simulink model "ISRTest2"  (Simulink 6.6)
settings: Solver=ode3  StartTime=0.0  StopTime=time(end)  FixedStep=0.01  RelTol=1e-3
values from neighbouring files (symbols this model uses):
  apSampleTime = 0.01    [Load_Replay.m]    (also in loadReplayMay2013.m; loadTuneRollReplay_May2013.m; replayFlight.m)
  bankCommandLimit = single(45*pi/180)    [replayFlight.m]
  ISA_g = 9.815    [replayFlight.m]
undefined symbols (not defined in the file or in its folder): fOrderingInOut, maxAcc, maxEta
libraries: simulink x14, aerolibconvert2 x11, dsPICdrivers x7, SLUGS_Library x3, dspmtrx3 x2, aerolibutil x1
(part 1 of 2)
settings Model: Creator=Administrator  LastModifiedBy=Administrator

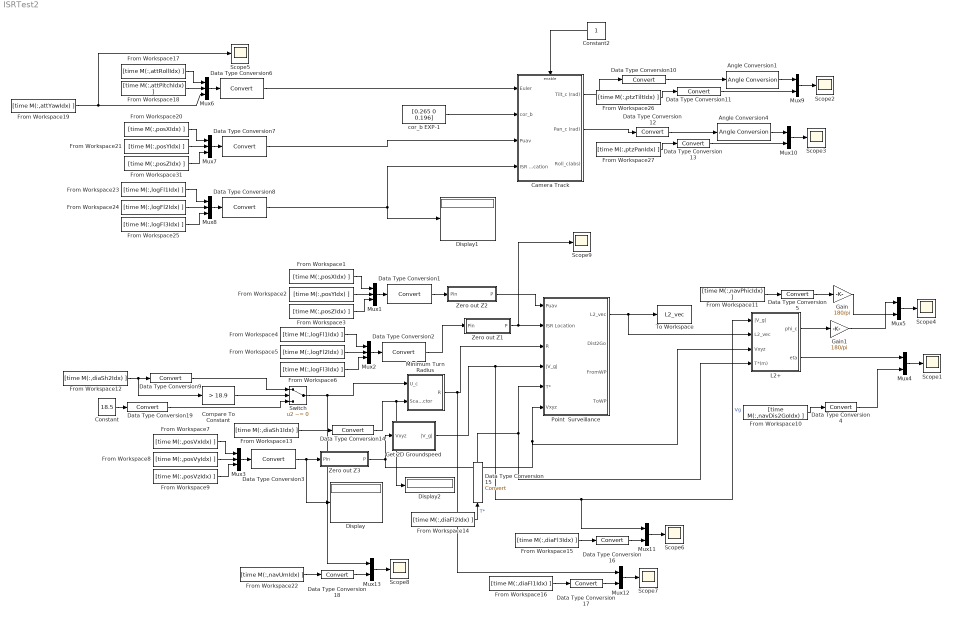
== system ISRTest2 ==
  Angle Conversion1 : aerolibconvert2/Angle Conversion  SystemSampleTime=-1  IU=rad  OU=deg
  Angle Conversion4 : aerolibconvert2/Angle Conversion  SystemSampleTime=-1  IU=rad  OU=deg
  Camera Track : Subsystem  TreatAsAtomicUnit=on  SystemSampleTime=0.01
  Compare To Constant : simulink/Logic and Bit Operations/Compare To Constant  SystemSampleTime=-1  relop=>  const=18.9  LogicOutDataTypeMode=uint8  ZeroCross=off
  Constant : Constant  Value=18.5
  Constant2 : Constant  Orientation=left  OutDataTypeMode=uint8
  Data Type Conversion{1..14,16..19} (18 alike) : DataTypeConversion  OutDataTypeMode=single
  Data Type Conversion15 : DataTypeConversion  Orientation=up  OutDataTypeMode=single
  Display : Display
  Display1 : Display
  Display2 : Display
  From Workspace1 : FromWorkspace  VariableName=[time M(:,posXIdx) ]  SampleTime=0.01
  From Workspace10 : FromWorkspace  VariableName=[time M(:,navDis2GoIdx) ]  SampleTime=0.01
  From Workspace11 : FromWorkspace  VariableName=[time M(:,navPhicIdx) ]  SampleTime=0.01
  From Workspace12 : FromWorkspace  VariableName=[time M(:,diaSh2Idx) ]  SampleTime=0.01
  From Workspace13 : FromWorkspace  VariableName=[time M(:,diaSh1Idx) ]  SampleTime=0.01
  From Workspace14 : FromWorkspace  VariableName=[time M(:,diaFl2Idx) ]  SampleTime=0.01
  From Workspace15 : FromWorkspace  VariableName=[time M(:,diaFl3Idx) ]  SampleTime=0.01
  From Workspace16 : FromWorkspace  VariableName=[time M(:,diaFl1Idx) ]  SampleTime=0.01
  From Workspace17 : FromWorkspace  VariableName=[time M(:,attRollIdx) ]  SampleTime=0.01
  From Workspace18 : FromWorkspace  VariableName=[time M(:,attPitchIdx) ]  SampleTime=0.01
  From Workspace19 : FromWorkspace  VariableName=[time M(:,attYawIdx) ]  SampleTime=0.01
  From Workspace2 : FromWorkspace  VariableName=[time M(:,posYIdx) ]  SampleTime=0.01
  From Workspace20 : FromWorkspace  VariableName=[time M(:,posXIdx) ]  SampleTime=0.01
  From Workspace21 : FromWorkspace  VariableName=[time M(:,posYIdx) ]  SampleTime=0.01
  From Workspace22 : FromWorkspace  VariableName=[time M(:,navUmIdx) ]  SampleTime=0.01
  From Workspace23 : FromWorkspace  VariableName=[time M(:,logFl1Idx) ]  SampleTime=0.01
  From Workspace24 : FromWorkspace  VariableName=[time M(:,logFl2Idx) ]  SampleTime=0.01
  From Workspace25 : FromWorkspace  VariableName=[time M(:,logFl3Idx) ]  SampleTime=0.01
  From Workspace26 : FromWorkspace  VariableName=[time M(:,ptzTiltIdx) ]  SampleTime=0.01
  From Workspace27 : FromWorkspace  VariableName=[time M(:,ptzPanIdx) ]  SampleTime=0.01
  From Workspace3 : FromWorkspace  VariableName=[time M(:,posZIdx) ]  SampleTime=0.01
  From Workspace31 : FromWorkspace  VariableName=[time M(:,posZIdx) ]  SampleTime=0.01
  From Workspace4 : FromWorkspace  VariableName=[time M(:,logFl1Idx) ]  SampleTime=0.01
  From Workspace5 : FromWorkspace  VariableName=[time M(:,logFl2Idx) ]  SampleTime=0.01
  From Workspace6 : FromWorkspace  VariableName=[time M(:,logFl3Idx) ]  SampleTime=0.01
  From Workspace7 : FromWorkspace  VariableName=[time M(:,posVxIdx) ]  SampleTime=0.01
  From Workspace8 : FromWorkspace  VariableName=[time M(:,posVyIdx) ]  SampleTime=0.01
  From Workspace9 : FromWorkspace  VariableName=[time M(:,posVzIdx) ]  SampleTime=0.01
  Gain : Gain  Gain=180/pi
  Gain1 : Gain  Gain=180/pi
  Get 2D Groundspeed : Subsystem
  L2+ : Subsystem
  Minimum Turn Radius : Subsystem
  Mux{1..3,6..8} (6 alike) : Mux  Inputs=3
  Mux{4..5,9..13} (7 alike) : Mux  Inputs=2
  Point  Surveillance : Subsystem  TreatAsAtomicUnit=on
  Scope{1..9} (9 alike) : Scope
      Scope1 settings: YMin=-120  YMax=30
      Scope2 settings: TimeRange=1267.6  YMin=-65  YMax=0  SaveName=ScopeData5
      Scope3 settings: TimeRange=600  YMin=49.80645682246021  YMax=134.5919948321196  SaveName=ScopeData6
      Scope4 settings: YMin=-15  YMax=25  SaveName=ScopeData7
      Scope5 settings: SaveName=ScopeData10
      Scope6 settings: TimeRange=600  YMin=12  YMax=24  SaveName=ScopeData11
      Scope7 settings: YMin=373  YMax=395  SaveName=ScopeData12
      Scope8 settings: YMin=17.75  YMax=20.25  SaveName=ScopeData13
      Scope9 settings: TimeRange=1429.39  YMin=-67.5  YMax=-27.5  SaveName=ScopeData19
  Switch : Switch  Criteria=u2 ~= 0  Threshold=0.3
  To Workspace : ToWorkspace  VariableName=L2_vec  SampleTime=-1  SaveFormat=Array
  Zero out Z1 : Stateflow chart
  Zero out Z2 : Stateflow chart
  Zero out Z3 : Stateflow chart
  cor_b EXP-1 : Constant  Value=[0.265 0 0.196]  OutDataTypeMode=single
  wires:
  Mux6/1 -> Data Type Conversion6/1
  From Workspace17/1 -> Mux6/1
  From Workspace18/1 -> Mux6/2
  From Workspace19/1 -> Mux6/3, Scope5/1
  Data Type Conversion6/1 -> Camera Track/1(Euler)
  cor_b EXP-1/1 -> Camera Track/2(cor_b)
  Mux7/1 -> Data Type Conversion7/1
  From Workspace20/1 -> Mux7/1
  From Workspace21/1 -> Mux7/2
  Data Type Conversion7/1 -> Camera Track/3(Puav)
  Mux8/1 -> Data Type Conversion8/1
  From Workspace23/1 -> Mux8/1
  From Workspace24/1 -> Mux8/2
  From Workspace25/1 -> Mux8/3
  Data Type Conversion8/1 -> Camera Track/4(ISR Location), Display1/1
  Constant2/1 -> Camera Track/Enable
  Mux9/1 -> Scope2/1
  Camera Track/1(Tilt_c (rad)) -> Data Type Conversion10/1
  From Workspace26/1 -> Data Type Conversion11/1
  Mux10/1 -> Scope3/1
  From Workspace27/1 -> Data Type Conversion13/1
  Camera Track/2(Pan_c (rad)) -> Data Type Conversion12/1
  Data Type Conversion10/1 -> Angle Conversion1/1
  Data Type Conversion11/1 -> Mux9/2
  Data Type Conversion12/1 -> Angle Conversion4/1
  Data Type Conversion13/1 -> Mux10/2
  From Workspace31/1 -> Mux7/3
  Angle Conversion4/1 -> Mux10/1
  Angle Conversion1/1 -> Mux9/1
  Mux1/1 -> Data Type Conversion1/1
  From Workspace1/1 -> Mux1/1
  From Workspace2/1 -> Mux1/2
  From Workspace3/1 -> Mux1/3
  Data Type Conversion1/1 -> Zero out Z2/1(Pin)
  Zero out Z2/1(P) -> Point  Surveillance/1(Puav)
  Mux2/1 -> Data Type Conversion2/1
  From Workspace4/1 -> Mux2/1
  From Workspace5/1 -> Mux2/2
  From Workspace6/1 -> Mux2/3
  Data Type Conversion2/1 -> Zero out Z1/1(Pin)
  Zero out Z1/1(P) -> Point  Surveillance/2(ISR Location), Scope9/1
  Minimum Turn Radius/1(R) -> Point  Surveillance/3(R), Mux12/1
  From Workspace12/1 -> Data Type Conversion9/1, Compare To Constant/1
  From Workspace13/1 -> Data Type Conversion14/1
  Zero out Z3/1(P) -> Get 2D Groundspeed/1(Vxyz), L2+/3(Vxyz), Point  Surveillance/6(Vxyz)
  Get 2D Groundspeed/1(|V_g|) -> Point  Surveillance/4(|V_g|), L2+/1(|V_g|), Mux11/1  "Vg"
  Mux3/1 -> Data Type Conversion3/1
  From Workspace7/1 -> Mux3/1
  From Workspace8/1 -> Mux3/2
  From Workspace9/1 -> Mux3/3
  Data Type Conversion3/1 -> Zero out Z3/1(Pin), Display/1
  From Workspace14/1 -> Data Type Conversion15/1  "T*"
  Point  Surveillance/1(L2_vec) -> To Workspace/1, L2+/2(L2_vec)
  L2+/2(eta) -> Mux4/1
  Mux4/1 -> Scope1/1
  From Workspace10/1 -> Data Type Conversion4/1
  Data Type Conversion4/1 -> Mux4/2
  Mux5/1 -> Scope4/1
  From Workspace11/1 -> Data Type Conversion5/1
  Data Type Conversion5/1 -> Gain/1
  L2+/1(phi_c) -> Gain1/1
  Data Type Conversion14/1 -> Minimum Turn Radius/2(Scale Factor), Display2/1
  Data Type Conversion15/1 -> L2+/4(T*(m)), Point  Surveillance/5(T*)
  Gain/1 -> Mux5/2
  Gain1/1 -> Mux5/1
  Mux11/1 -> Scope6/1
  From Workspace15/1 -> Data Type Conversion16/1
  Data Type Conversion16/1 -> Mux11/2
  Mux12/1 -> Scope7/1
  From Workspace16/1 -> Data Type Conversion17/1
  Data Type Conversion17/1 -> Mux12/2
  From Workspace22/1 -> Data Type Conversion18/1
  Data Type Conversion18/1 -> Mux13/2
  Mux13/1 -> Scope8/1
  Switch/1 -> Minimum Turn Radius/1(U_c), Mux13/1
  Data Type Conversion9/1 -> Switch/1
  Compare To Constant/1 -> Switch/2
  Constant/1 -> Data Type Conversion19/1
  Data Type Conversion19/1 -> Switch/3

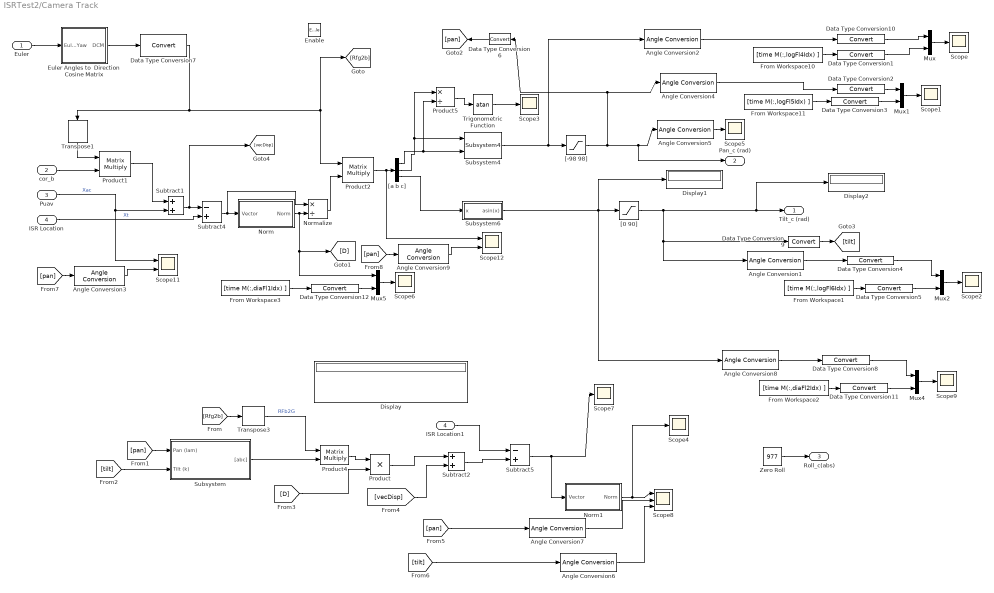
== system ISRTest2/Camera Track ==
  Euler : Inport
  cor_b : Inport  Port=2
  Puav : Inport  Port=3
  ISR Location : Inport  Port=4
  Enable : EnablePort
  Angle Conversion{1..9} (9 alike) : aerolibconvert2/Angle Conversion  SystemSampleTime=-1  IU=rad  OU=deg
  Data Type Conversion{1..5,7..12} (11 alike) : DataTypeConversion  OutDataTypeMode=single
  Data Type Conversion6 : DataTypeConversion  Orientation=left  OutDataTypeMode=single
  Display : Display
  Display1 : Display
  Display2 : Display
  Euler Angles to  Direction Cosine Matrix : Subsystem  AncestorBlock="aerolibtransform2/Euler Angles to  Direction Cosine Matrix"  mask(Euler2DCM){}
      mask help: Determine the 3-by-3 direction cosine matrix (DCM) from an Euler orientation (roll, pitch, yaw). The output DCM transforms vectors from geodetic earth or north-east-down (NED) axes to body axes.
      mask init:
      | aeroicon('aeroblk');
      mask Help: web(asbhelp('euleranglestodirectioncosinematrix'));
      mask Display:
      | port_label('input',1,'\phi \theta \psi','texmode','on')
      | port_label('output',1,'DCM_{be}','texmode','on')
  From Workspace1 : FromWorkspace  VariableName=[time M(:,logFl6Idx) ]  SampleTime=0.01
  From Workspace10 : FromWorkspace  VariableName=[time M(:,logFl4Idx) ]  SampleTime=0.01
  From Workspace11 : FromWorkspace  VariableName=[time M(:,logFl5Idx) ]  SampleTime=0.01
  From Workspace2 : FromWorkspace  VariableName=[time M(:,diaFl2Idx) ]  SampleTime=0.01
  From Workspace3 : FromWorkspace  VariableName=[time M(:,diaFl1Idx) ]  SampleTime=0.01
  ISR Location1 : InportShadow  Port=4  LatchByCopyingInsideSignal=off
  Mux{,1..2,4..5} (5 alike) : Mux  Inputs=2
  Norm : Subsystem
  Norm1 : Subsystem
  Normalize : Product  Inputs=*/  OutScaling=2^-10
  Product : Product  RndMeth=Zero
  Product1 : Product  Multiplication=Matrix(*)  RndMeth=Zero
  Product2 : Product  Multiplication=Matrix(*)  RndMeth=Zero
  Product4 : Product  Multiplication=Matrix(*)  RndMeth=Zero
  Product5 : Product  Inputs=*/  RndMeth=Zero
  Scope{,1..7,9} (9 alike) : Scope
      Scope settings: YMin=20  YMax=170  SaveName=ScopeData2
      Scope1 settings: SaveName=ScopeData3
      Scope2 settings: SaveName=ScopeData4
      Scope3 settings: YMin=-1.75  YMax=1.75  SaveName=ScopeData8
      Scope4 settings: YMin=0  YMax=75
      Scope5 settings: YMin=-90  YMax=90  SaveName=ScopeData14
      Scope6 settings: YMin=-90  YMax=90  SaveName=ScopeData15
      Scope7 settings: YMin=-90  YMax=90  SaveName=ScopeData16
      Scope9 settings: SaveName=ScopeData18
  Scope11 : Scope  NumInputPorts=2
      settings: YMin=-125~-100  YMax=175~100  SaveName=ScopeData20
  Scope12 : Scope  NumInputPorts=2
      settings: YMin=-1~-57.5  YMax=0.4~-20  SaveName=ScopeData21
  Scope8 : Scope  NumInputPorts=3
      settings: YMin=0~-100~57.5  YMax=110~100~90  SaveName=ScopeData17
  Subsystem : Subsystem
  Subsystem4 : SLUGS_Library/Subsystem4  SystemSampleTime=-1
  Subsystem6 : Subsystem  AncestorBlock=SLUGS_Library/Subsystem6
  Subtract1 : Sum  OutScaling=2^-10
  Subtract2 : Sum  OutScaling=2^-10
  Subtract4 : Sum  Inputs=-+  OutScaling=2^-10
  Subtract5 : Sum  Inputs=-+  OutScaling=2^-10
  Transpose1 : dspmtrx3/Transpose  Orientation=down  SystemSampleTime=-1  Hermitian=off  overflowFlag=off
  Transpose3 : dspmtrx3/Transpose  SystemSampleTime=-1  Hermitian=off  overflowFlag=off
  Trigonometric Function : Trigonometry  Operator=atan
  Zero Roll : Constant  Value=977  OutDataTypeMode=uint16
  "[-98 98]" : Saturate  UpperLimit=1.7104  LowerLimit=-1.7104
  "[0 90]" : Saturate  UpperLimit=0  LowerLimit=-pi/2
  "[a b c]" : Demux  Outputs=3
  Tilt_c (rad) : Outport
  Pan_c (rad) : Outport  Port=2
  Roll_c(abs) : Outport  Port=3  InitialOutput=977
  wires:
  Angle Conversion1/1 -> Data Type Conversion4/1
  Angle Conversion2/1 -> Data Type Conversion10/1
  Zero Roll/1 -> Roll_c(abs)/1
  cor_b/1 -> Product1/2
  Norm/1(Norm) -> Normalize/2, [D], Mux5/1
  Normalize/1 -> Product2/2
  Product2/1 -> "[a b c]"/1, Scope12/1
  "[a b c]"/3 -> Subsystem6/1(x)
  "[a b c]"/2 -> Subsystem4/1, Product5/1
  "[a b c]"/1 -> Subsystem4/2, Product5/2
  Subtract4/1 -> Norm/1(Vector), Normalize/1
  "[0 90]"/1 -> Angle Conversion1/1, Data Type Conversion9/1, Tilt_c (rad)/1, Display2/1
  Mux/1 -> Scope/1
  From Workspace10/1 -> Data Type Conversion1/1
  Mux1/1 -> Scope1/1
  Angle Conversion4/1 -> Data Type Conversion2/1
  From Workspace11/1 -> Data Type Conversion3/1
  Mux2/1 -> Scope2/1
  From Workspace1/1 -> Data Type Conversion5/1
  Data Type Conversion10/1 -> Mux/1
  Data Type Conversion1/1 -> Mux/2
  Data Type Conversion2/1 -> Mux1/1
  Data Type Conversion3/1 -> Mux1/2
  Data Type Conversion4/1 -> Mux2/1
  Data Type Conversion5/1 -> Mux2/2
  Transpose1/1 -> Product1/1
  Subtract1/1 -> Subtract4/1, [vecDisp]
  ISR Location/1 -> Subtract4/2  "Xt"
  Product1/1 -> Subtract1/1
  Puav/1 -> Subtract1/2, Scope11/1  "Xac"
  Subsystem4/1 -> "[-98 98]"/1, Angle Conversion2/1
  Angle Conversion5/1 -> Scope5/1
  "[-98 98]"/1 -> Data Type Conversion6/1, Angle Conversion4/1, Angle Conversion5/1, Pan_c (rad)/1
  Data Type Conversion9/1 -> [tilt]
  Data Type Conversion6/1 -> [pan]
  [Rfg2b] -> Transpose3/1
  Subsystem/1("[abc]") -> Product4/2
  Transpose3/1 -> Product4/1  "RFb2G"
  [vecDisp] -> Subtract2/2
  Subtract2/1 -> Subtract5/2
  ISR Location1/1 -> Subtract5/1
  Subtract5/1 -> Scope7/1, Norm1/1(Vector)
  Norm1/1(Norm) -> Scope8/1, Scope4/1
  [pan] -> Angle Conversion7/1
  Angle Conversion7/1 -> Scope8/2
  Angle Conversion6/1 -> Scope8/3
  Euler Angles to  Direction Cosine Matrix/1(DCM) -> Data Type Conversion7/1
  Euler/1 -> Euler Angles to  Direction Cosine Matrix/1(Euler Roll Pitch Yaw)
  Data Type Conversion7/1 -> Transpose1/1, Product2/1, [Rfg2b]
  Subsystem6/1(asin(x)) -> Angle Conversion8/1, Display1/1, "[0 90]"/1
  Angle Conversion8/1 -> Data Type Conversion8/1
  Mux4/1 -> Scope9/1
  From Workspace2/1 -> Data Type Conversion11/1
  Data Type Conversion8/1 -> Mux4/1
  Data Type Conversion11/1 -> Mux4/2
  From Workspace3/1 -> Data Type Conversion12/1
  Data Type Conversion12/1 -> Mux5/2
  Mux5/1 -> Scope6/1
  Trigonometric Function/1 -> Scope3/1
  [pan] -> Angle Conversion3/1
  Angle Conversion3/1 -> Scope11/2
  [pan] -> Angle Conversion9/1
  Angle Conversion9/1 -> Scope12/2
  [tilt] -> Angle Conversion6/1
  Product5/1 -> Trigonometric Function/1
  Product4/1 -> Product/1
  [D] -> Product/2
  Product/1 -> Subtract2/1
  [pan] -> Subsystem/1(Pan (lam))
  [tilt] -> Subsystem/2(Tilt (k))

== system ISRTest2/Get 2D Groundspeed ==
  Vxyz : Inport  SampleTime=apSampleTime
  Norm : Subsystem
  |V_g| : Outport
  wires:
  Norm/1(Norm) -> |V_g|/1
  Vxyz/1 -> Norm/1(Vector)

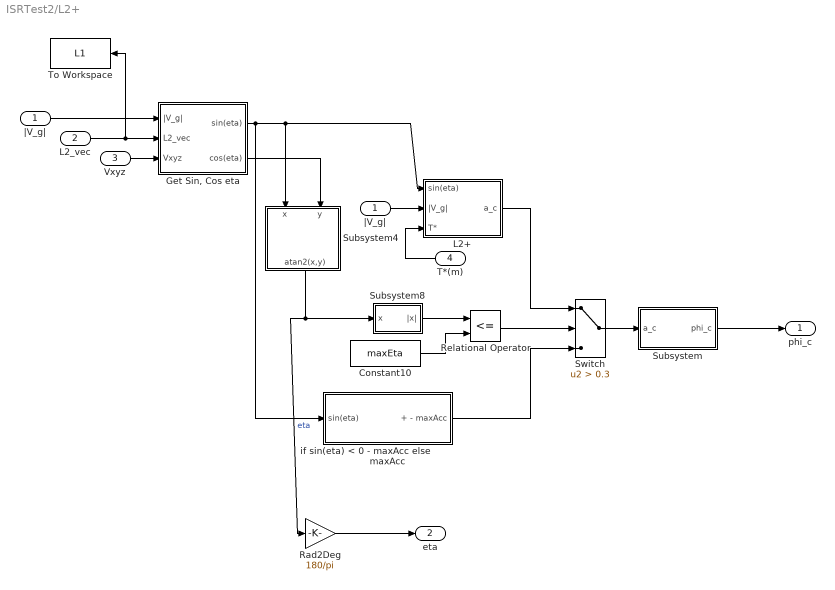
== system ISRTest2/L2+ ==
  |V_g| : Inport
  L2_vec : Inport  Port=2
  Vxyz : Inport  Port=3
  T*(m) : Inport  Orientation=left  Port=4
  Constant10 : Constant  Value=maxEta  OutDataTypeMode=single
  "Get Sin, Cos eta" : Subsystem
  L2+ : Subsystem
  Rad2Deg : Gain  Gain=180/pi
  Relational Operator : RelationalOperator  Operator=<=  LogicOutDataTypeMode=Boolean
  Subsystem : Subsystem
  Subsystem4 : Subsystem  Orientation=down
  Subsystem8 : Subsystem  AncestorBlock=SLUGS_Library/Subsystem8
  Switch : Switch  Criteria=u2 > Threshold  Threshold=0.3
  To Workspace : ToWorkspace  VariableName=L1  SampleTime=-1  SaveFormat=Array
  "if sin(eta) < 0 - maxAcc else                 maxAcc " : Subsystem
  "|V_g| " : InportShadow  Port=1  LatchByCopyingInsideSignal=off
  phi_c : Outport
  eta : Outport  Port=2
  wires:
  Rad2Deg/1 -> eta/1
  Subsystem/1(phi_c) -> phi_c/1
  T*(m)/1 -> L2+/3(T*)
  "|V_g| "/1 -> L2+/2(|V_g|)
  "Get Sin, Cos eta"/1(sin(eta)) -> L2+/1(sin(eta)), Subsystem4/1(x), "if sin(eta) < 0 - maxAcc else                 maxAcc "/1(sin(eta))
  "Get Sin, Cos eta"/2(cos(eta)) -> Subsystem4/2(y)
  Subsystem4/1(atan2(x,y)) -> Rad2Deg/1, Subsystem8/1(x)  "eta"
  Subsystem8/1(|x|) -> Relational Operator/1
  Constant10/1 -> Relational Operator/2
  Relational Operator/1 -> Switch/2
  L2+/1(a_c) -> Switch/1
  "if sin(eta) < 0 - maxAcc else                 maxAcc "/1(+ - maxAcc) -> Switch/3
  Switch/1 -> Subsystem/1(a_c)
  |V_g|/1 -> "Get Sin, Cos eta"/1(|V_g|)
  L2_vec/1 -> To Workspace/1, "Get Sin, Cos eta"/2(L2_vec)
  Vxyz/1 -> "Get Sin, Cos eta"/3(Vxyz)

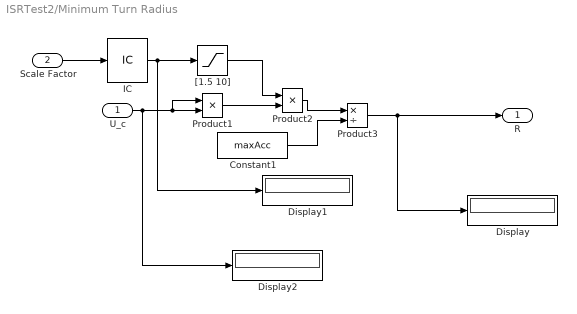
== system ISRTest2/Minimum Turn Radius ==
  U_c : Inport
  Scale Factor : Inport  Port=2
  Constant1 : Constant  Value=maxAcc  OutDataTypeMode=single
  Display : Display
  Display1 : Display
  Display2 : Display
  IC : InitialCondition  Value=1.5
  Product1 : Product  RndMeth=Zero
  Product2 : Product  RndMeth=Zero
  Product3 : Product  Inputs=*/  RndMeth=Zero
  "[1.5 10]" : Saturate  UpperLimit=10  LowerLimit=1.5
  R : Outport
  wires:
  IC/1 -> "[1.5 10]"/1, Display1/1
  "[1.5 10]"/1 -> Product2/1
  Product3/1 -> R/1, Display/1
  Scale Factor/1 -> IC/1
  Product1/1 -> Product2/2
  Constant1/1 -> Product3/2
  Product2/1 -> Product3/1
  U_c/1 -> Product1/1, Product1/2, Display2/1

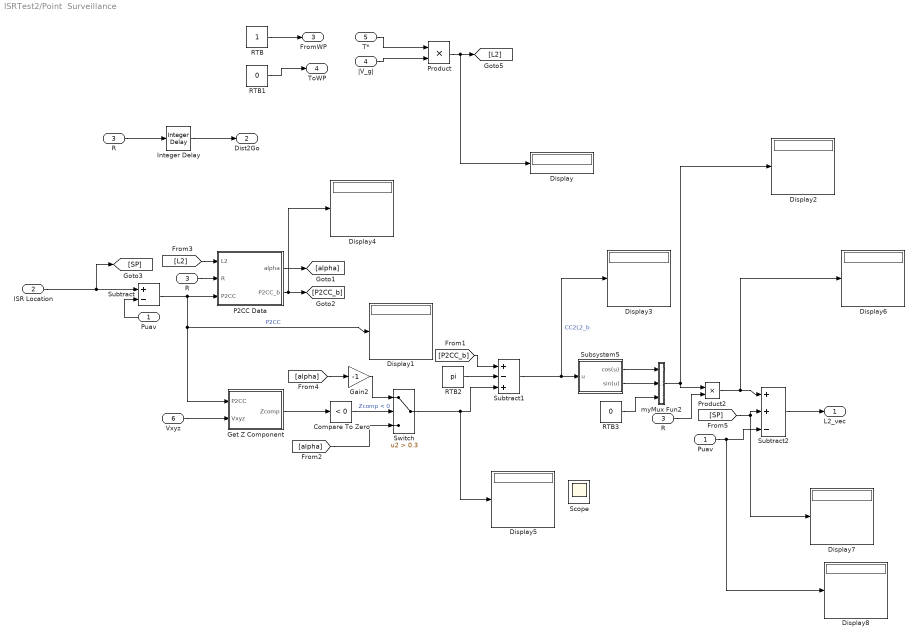
== system ISRTest2/Point  Surveillance ==
  Puav : Inport  Orientation=left
  ISR Location : Inport  Port=2
  R : Inport  Port=3
  |V_g| : Inport  Port=4
  T* : Inport  Port=5
  Vxyz : Inport  Port=6
  Compare To Zero : simulink/Logic and Bit Operations/Compare To Zero  SystemSampleTime=-1  relop=<  LogicOutDataTypeMode=uint8  ZeroCross=off
  Display{,1..8} (9 alike) : Display
  Gain2 : Gain  Gain=-1
  Get Z Component : Subsystem
  Integer Delay : simulink/Discrete/Integer Delay  vinit=0.0  samptime=-1  NumDelays=1
  P2CC Data : Subsystem
  Product : Product  OutDataTypeMode=single  RndMeth=Zero
  Product2 : Product  RndMeth=Zero
  "Puav  " : InportShadow  Port=1  LatchByCopyingInsideSignal=off
  "R " : InportShadow  Port=3  LatchByCopyingInsideSignal=off
  "R  " : InportShadow  Port=3  LatchByCopyingInsideSignal=off
  RTB : Constant  OutDataTypeMode=uint8  SampleTime=0.01
  RTB1 : Constant  Value=0  OutDataTypeMode=uint8  SampleTime=0.01
  RTB2 : Constant  Value=pi  OutDataTypeMode=single
  RTB3 : Constant  Value=0  OutDataTypeMode=single
  Scope : Scope  NumInputPorts=4
      settings: YMin=-5~-5~-5~-5  YMax=5~5~5~5  SaveName=ScopeData9
  Subsystem5 : Subsystem
  Subtract : Sum  Inputs=+-  OutScaling=2^-10
  Subtract1 : Sum  Inputs=+-+  OutScaling=2^-10
  Subtract2 : Sum  Inputs=++-  OutScaling=2^-10
  Switch : Switch  Criteria=u2 > Threshold  Threshold=0.3  ZeroCross=off
  myMux Fun2 : Stateflow chart
  L2_vec : Outport
  Dist2Go : Outport  Port=2
  FromWP : Outport  Port=3  InitialOutput=[1]
  ToWP : Outport  Port=4  InitialOutput=[1]
  wires:
  "R  "/1 -> Integer Delay/1
  Subtract2/1 -> L2_vec/1
  "Puav  "/1 -> Subtract2/3, Display8/1
  [SP] -> Subtract2/2, Display7/1
  Product2/1 -> Subtract2/1, Display6/1
  "R "/1 -> Product2/2
  myMux Fun2/1(y) -> Product2/1, Display2/1
  RTB3/1 -> myMux Fun2/3(u3)
  Subsystem5/2(sin(u)) -> myMux Fun2/2(u2)
  Subsystem5/1(cos(u)) -> myMux Fun2/1(u1)
  Subtract1/1 -> Subsystem5/1(u), Display3/1  "CC2L2_b"
  Switch/1 -> Subtract1/3, Display5/1
  Gain2/1 -> Switch/1
  [alpha] -> Gain2/1
  [alpha] -> Switch/3
  RTB2/1 -> Subtract1/2
  [P2CC_b] -> Subtract1/1
  [L2] -> P2CC Data/1(L2)
  Compare To Zero/1 -> Switch/2  "Zcomp < 0"
  Get Z Component/1(Zcomp) -> Compare To Zero/1
  P2CC Data/1(alpha) -> [alpha]
  P2CC Data/2(P2CC_b) -> [P2CC_b], Display4/1
  Vxyz/1 -> Get Z Component/2(Vxyz)
  R/1 -> P2CC Data/2(R)
  Subtract/1 -> P2CC Data/3(P2CC), Get Z Component/1(P2CC), Display1/1  "P2CC"
  Puav/1 -> Subtract/2
  ISR Location/1 -> [SP], Subtract/1
  Product/1 -> [L2], Display/1
  |V_g|/1 -> Product/2
  T*/1 -> Product/1
  RTB1/1 -> ToWP/1
  RTB/1 -> FromWP/1
  Integer Delay/1 -> Dist2Go/1

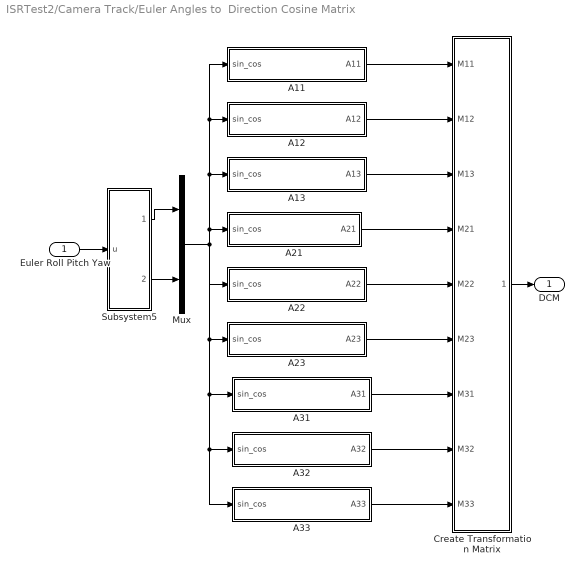
== system ISRTest2/Camera Track/Euler Angles to  Direction Cosine Matrix ==
  Euler Roll Pitch Yaw : Inport  PortDimensions=3
  A11 : Subsystem
  A12 : Subsystem
  A13 : Subsystem
  A21 : Subsystem
  A22 : Subsystem
  A23 : Subsystem
  A31 : Subsystem
  A32 : Subsystem
  A33 : Subsystem
  Create Transformation Matrix : Subsystem  AncestorBlock=aerolibutil/Create 3x3 Matrix  mask(Create 3x3 Matrix){}
      mask help:
      | Create a 3-by-3 matrix from nine input values. Each input corresponds to an element of the matrix.
      |
      | For example, the input labeled A21 is the entry in the second row and first column of the matrix.
      mask init:
      | aeroicon('aeroblk');
      mask Help: web(asbhelp);
      mask Display:
      | port_label('input',1,'A_{11}','texmode','on');
      | port_label('input',2,'A_{12}','texmode','on');
      | port_label('input',3,'A_{13}','texmode','on');
      | port_label('input',4,'A_{21}','texmode','on');
      | port_label('input',5,'A_{22}','texmode','on');
      | port_label('input',6,'A_{23}','texmode','on');
      | port_label('input',7,'A_{31}','texmode','on');
      | port_label('input',8,'A_{32}','texmode','on');
      | port_label('input',9,'A_{33}','texmode','on');
      | port_label('output',1,'A','texmode','on');
  Mux : Mux  Inputs=2
  Subsystem5 : Subsystem  AncestorBlock=SLUGS_Library/Subsystem5
  DCM : Outport  PortDimensions=[3,3]  InitialOutput=0
  wires:
  A13/1(A13) -> Create Transformation Matrix/3(M13)
  A22/1(A22) -> Create Transformation Matrix/5(M22)
  A11/1(A11) -> Create Transformation Matrix/1(M11)
  A12/1(A12) -> Create Transformation Matrix/2(M12)
  A23/1(A23) -> Create Transformation Matrix/6(M23)
  A33/1(A33) -> Create Transformation Matrix/9(M33)
  A32/1(A32) -> Create Transformation Matrix/8(M32)
  A31/1(A31) -> Create Transformation Matrix/7(M31)
  A21/1(A21) -> Create Transformation Matrix/4(M21)
  Create Transformation Matrix/1(Matrix) -> DCM/1
  Subsystem5/1(sin(u)) -> Mux/1
  Subsystem5/2(cos(u)) -> Mux/2
  Euler Roll Pitch Yaw/1 -> Subsystem5/1(u)
  Mux/1 -> A22/1(sin_cos), A21/1(sin_cos), A12/1(sin_cos), A11/1(sin_cos), A13/1(sin_cos), A23/1(sin_cos), A31/1(sin_cos), A32/1(sin_cos), A33/1(sin_cos)

== system ISRTest2/Camera Track/Norm ==
  Vector : Inport
  Subsystem1 : Subsystem  AncestorBlock=SLUGS_Library/Subsystem1
  Subsystem3 : Subsystem  AncestorBlock=SLUGS_Library/Subsystem3
  Norm : Outport
  wires:
  Subsystem1/1(sqrt(x)) -> Norm/1
  Vector/1 -> Subsystem3/1(x), Subsystem3/2(y)
  Subsystem3/1(x dot y) -> Subsystem1/1(x)

== system ISRTest2/Camera Track/Norm1 ==
  Vector : Inport
  Subsystem1 : Subsystem  AncestorBlock=SLUGS_Library/Subsystem1
  Subsystem3 : Subsystem  AncestorBlock=SLUGS_Library/Subsystem3
  Norm : Outport
  wires:
  Subsystem3/1(x dot y) -> Subsystem1/1(x)
  Vector/1 -> Subsystem3/2(y), Subsystem3/1(x)
  Subsystem1/1(sqrt(x)) -> Norm/1

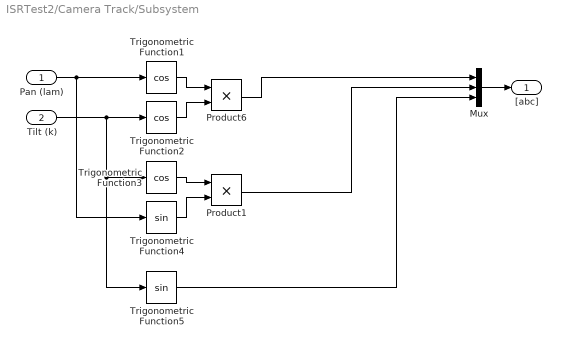
== system ISRTest2/Camera Track/Subsystem ==
  Pan (lam) : Inport
  Tilt (k) : Inport  Port=2
  Mux : Mux  Inputs=3
  Product1 : Product  RndMeth=Zero
  Product6 : Product  RndMeth=Zero
  Trigonometric Function1 : Trigonometry  Operator=cos
  Trigonometric Function2 : Trigonometry  Operator=cos
  Trigonometric Function3 : Trigonometry  Operator=cos
  Trigonometric Function4 : Trigonometry
  Trigonometric Function5 : Trigonometry
  "[abc]" : Outport
  wires:
  Trigonometric Function1/1 -> Product6/1
  Trigonometric Function2/1 -> Product6/2
  Pan (lam)/1 -> Trigonometric Function1/1, Trigonometric Function4/1
  Tilt (k)/1 -> Trigonometric Function2/1, Trigonometric Function3/1, Trigonometric Function5/1
  Mux/1 -> "[abc]"/1
  Product6/1 -> Mux/1
  Trigonometric Function3/1 -> Product1/1
  Trigonometric Function4/1 -> Product1/2
  Product1/1 -> Mux/2
  Trigonometric Function5/1 -> Mux/3

== system ISRTest2/Camera Track/Subsystem6 ==
  x : Inport
  Trigonometric Function : Trigonometry  Operator=asin
  "[-1,1]" : Saturate  UpperLimit=0.9999  LowerLimit=-0.999
  asin(x) : Outport
  wires:
  "[-1,1]"/1 -> Trigonometric Function/1
  x/1 -> "[-1,1]"/1
  Trigonometric Function/1 -> asin(x)/1

== system ISRTest2/Get 2D Groundspeed/Norm ==
  Vector : Inport
  Subsystem1 : Subsystem  AncestorBlock=SLUGS_Library/Subsystem1
  Subsystem3 : SLUGS_Library/Subsystem3  SystemSampleTime=-1
  Norm : Outport
  wires:
  Subsystem3/1 -> Subsystem1/1(x)
  Vector/1 -> Subsystem3/2, Subsystem3/1
  Subsystem1/1(sqrt(x)) -> Norm/1

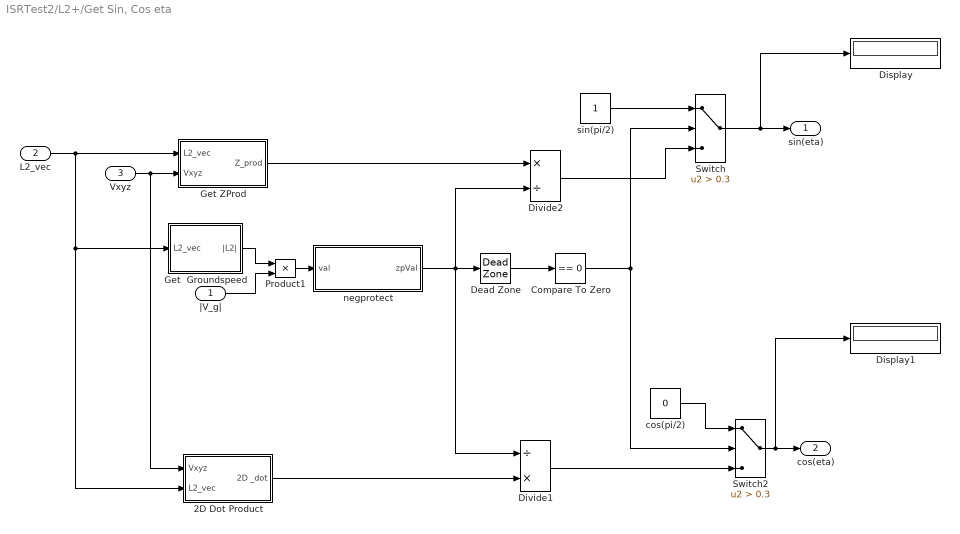
== system ISRTest2/L2+/Get Sin, Cos eta ==
  |V_g| : Inport
  L2_vec : Inport  Port=2
  Vxyz : Inport  Port=3
  "2D Dot Product " : Subsystem
  Compare To Zero : simulink/Logic and Bit Operations/Compare To Zero  SystemSampleTime=-1  relop===  LogicOutDataTypeMode=uint8  ZeroCross=off
  Dead Zone : DeadZone  LowerValue=-0.1  UpperValue=0.1  SaturateOnIntegerOverflow=on
  Display : Display
  Display1 : Display
  Divide1 : Product  Inputs=/*  OutScaling=2^-10
  Divide2 : Product  Inputs=*/  OutScaling=2^-10
  Get  Groundspeed : Subsystem
  Get ZProd : Subsystem
  Product1 : Product  RndMeth=Zero
  Switch : Switch  Criteria=u2 > Threshold  Threshold=0.3  ZeroCross=off
  Switch2 : Switch  Criteria=u2 > Threshold  Threshold=0.3  ZeroCross=off
  cos(pi/2) : Constant  Value=0  OutDataTypeMode=single
  negprotect : Stateflow chart
  sin(pi/2) : Constant  OutDataTypeMode=single
  sin(eta) : Outport
  cos(eta) : Outport  Port=2
  wires:
  Compare To Zero/1 -> Switch/2, Switch2/2
  Dead Zone/1 -> Compare To Zero/1
  L2_vec/1 -> Get ZProd/1(L2_vec), "2D Dot Product "/2(L2_vec), Get  Groundspeed/1(L2_vec)
  Vxyz/1 -> Get ZProd/2(Vxyz), "2D Dot Product "/1(Vxyz)
  Get  Groundspeed/1(|L2|) -> Product1/1
  |V_g|/1 -> Product1/2
  Product1/1 -> negprotect/1(val)
  "2D Dot Product "/1(2D _dot) -> Divide1/2
  sin(pi/2)/1 -> Switch/1
  Switch2/1 -> cos(eta)/1, Display1/1
  cos(pi/2)/1 -> Switch2/1
  Divide1/1 -> Switch2/3
  Get ZProd/1(Z_prod) -> Divide2/1
  Divide2/1 -> Switch/3
  Switch/1 -> sin(eta)/1, Display/1
  negprotect/1(zpVal) -> Dead Zone/1, Divide1/1, Divide2/2

== system ISRTest2/L2+/L2+ ==
  sin(eta) : Inport
  |V_g| : Inport  Port=2
  T* : Inport  Port=3
  Display3 : Display
  Divide : Product  Inputs=**/  OutScaling=2^-10
  Gain : Gain  Gain=2  SampleTime=0.01
  negprotect : Stateflow chart
  a_c : Outport
  wires:
  negprotect/1(zpVal) -> Divide/3
  sin(eta)/1 -> Divide/1
  Divide/1 -> Gain/1
  |V_g|/1 -> Divide/2
  Gain/1 -> a_c/1, Display3/1
  T*/1 -> negprotect/1(val)

== system ISRTest2/L2+/Subsystem ==
  a_c : Inport
  Bank  Limit Command : Saturate  UpperLimit=bankCommandLimit  LowerLimit=-bankCommandLimit  SampleTime=apSampleTime
  Constant : Constant  Orientation=left  Value=ISA_g  OutDataTypeMode=single
  Product : Product  Inputs=*/  RndMeth=Zero
  Subsystem2 : Subsystem
  To Workspace3 : ToWorkspace  VariableName=Phic  SampleTime=-1  SaveFormat=Array
  phi_c : Outport
  wires:
  a_c/1 -> Product/1
  Constant/1 -> Product/2
  Product/1 -> Subsystem2/1(x)
  Subsystem2/1(atan(x)) -> Bank  Limit Command/1
  Bank  Limit Command/1 -> phi_c/1, To Workspace3/1

== system ISRTest2/L2+/Subsystem4 ==
  x : Inport
  y : Inport  Port=2
  C Function Call : S-Function  Tag=dsPIC_dsPIC_CFunctionCall  FunctionName=dsPIC_C_function_Call  Parameters=INPUT_SIZE,OUTPUT_SIZE,InputType,OutputType,SampleTime,fOrderingInOut  mask(C Function Call){fctName='myAtan2', INPUT_SIZE=1, INPUT1=real32, INPUT2=real32, INPUT3=--, OUTPUT_SIZE=1, OUTPUT1=real32, SampleTime=-1, InputType=[ 7 7 ], OutputType=[ 7 ], FctDeclaration=extern real32_T myAtan2(real32_T u1, real32_T u2);, FctCall=%y1 = myAtan2(%u1, %u2);, OrderingInOutPopup=None}
      mask prompts: fctName "Function Name"; INPUT_SIZE "Global Input Size"; INPUT1 "Input 1"; INPUT2 "Input 2"; INPUT3 "Input 3"; OUTPUT_SIZE "Output size"; OUTPUT1 "Output type"; InputType "NbrInput"; OutputType "NbrOutput"; FctDeclaration "Function Declaration :"; FctCall "Function Call :"; OrderingInOutPopup "Block Ordering Input / Output"
      mask help: call user defined C function
      mask init:
      | dsPIC_C_function_Call_callback();
      mask Help: http://www.kerhuel.eu/wiki/index.php5?title=Block/C_Function_Call#1
      mask StyleString: edit,edit,popup(--|int8|uint8|int16|uint16|int32|uint32|real32|real64),popup(--|int8|uint8|int16|uint16|int32|uint32|real32|real64),popup(--|int8|uint8|int16|uint16|int32|uint32|real32|real64),edit,popup(--|int8|uint8|int16|uint16|int32|uint32|real32|real64),edit,edit,edit,edit,edit,popup(None|Input|Output|Input & Output)
      mask CallbackString:
      | dsPIC_C_function_Call_callback();|dsPIC_C_function_Call_callback();|dsPIC_C_function_Call_callback();|dsPIC_C_function_Call_callback();
      | |dsPIC_C_function_Call_callback();|dsPIC_C_function_Call_callback();|dsPIC_C_function_Call_callback();|dsPIC_C_function_Call_callback();|||% for information only|% for information only|
      mask Display:
      | fprintf('C function call\nmyAtan2');
      | port_label('input',1,' u1');
      | port_label('input',2,' u2');
      | port_label('output',1,'y');
  Environment Controller : Subsystem  mask(Environment Controller){}
      mask help: Output the simulation (Sim) or Real-Time Workshop (RTW) port depending on the current environment. With optimizations enabled, unnecessary blocks leading to the unused port are not executed. Both input signals must be the same width.
      mask init:
      | switch_mode = rtwenvironmentmode(bdroot(gcbh));
  Trigonometric Function : Trigonometry  Operator=atan2
  atan2(x,y) : Outport
  wires:
  Environment Controller/1(Out) -> atan2(x,y)/1
  C Function Call/1 -> Environment Controller/2(RTW)
  Trigonometric Function/1 -> Environment Controller/1(Sim)
  y/1 -> C Function Call/2, Trigonometric Function/2
  x/1 -> C Function Call/1, Trigonometric Function/1

== system ISRTest2/L2+/Subsystem8 ==
  x : Inport
  Abs : Abs
  C Function Call : dsPICdrivers/OTHERS/C Function Call  Tag=dsPIC_dsPIC_CFunctionCall  fctName='myAbs'  INPUT_SIZE=1  INPUT1=real32  INPUT2=--  INPUT3=--  OUTPUT_SIZE=1  OUTPUT1=real32  SampleTime=-1  InputType=[ 7 ]  OutputType=[ 7 ]  FctDeclaration=extern real32_T myAbs(real32_T u1);  FctCall=%y1 = myAbs(%u1);  OrderingInOutPopup=None
  Environment Controller : simulink/Signal Routing/Environment Controller  SystemSampleTime=-1
  |x| : Outport
  wires:
  Environment Controller/1 -> |x|/1
  C Function Call/1 -> Environment Controller/2
  Abs/1 -> Environment Controller/1
  x/1 -> C Function Call/1, Abs/1

== system ISRTest2/L2+/if sin(eta) < 0 - maxAcc else                 maxAcc  ==
  sin(eta) : Inport
  Compare To Zero : simulink/Logic and Bit Operations/Compare To Zero  SystemSampleTime=-1  relop=<  LogicOutDataTypeMode=uint8  ZeroCross=off
  Constant1 : Constant  Value=maxAcc  OutDataTypeMode=single
  Constant9 : Constant  Value=-maxAcc  OutDataTypeMode=single
  Switch1 : Switch  Criteria=u2 > Threshold  Threshold=0.3
  + - maxAcc : Outport
  wires:
  Compare To Zero/1 -> Switch1/2
  Constant9/1 -> Switch1/1
  Constant1/1 -> Switch1/3
  sin(eta)/1 -> Compare To Zero/1
  Switch1/1 -> + - maxAcc/1

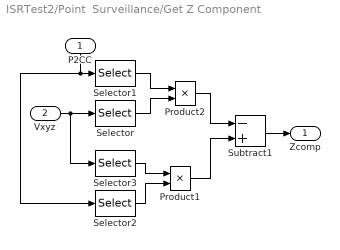
== system ISRTest2/Point  Surveillance/Get Z Component ==
  P2CC : Inport  Orientation=down
  Vxyz : Inport  Port=2
  Product1 : Product  RndMeth=Zero
  Product2 : Product  RndMeth=Zero
  Selector : Selector  IndexOptions=Index vector (dialog)  Indices=[2]  OutputSizes=1  InputPortWidth=3
  Selector1 : Selector  IndexOptions=Index vector (dialog)  Indices=[1]  OutputSizes=1  InputPortWidth=3
  Selector2 : Selector  IndexOptions=Index vector (dialog)  Indices=[2]  OutputSizes=1  InputPortWidth=3
  Selector3 : Selector  IndexOptions=Index vector (dialog)  Indices=[1]  OutputSizes=1  InputPortWidth=3
  Subtract1 : Sum  Inputs=-+  OutScaling=2^-10
  Zcomp : Outport
  wires:
  Subtract1/1 -> Zcomp/1
  P2CC/1 -> Selector2/1, Selector1/1
  Product1/1 -> Subtract1/2
  Product2/1 -> Subtract1/1
  Selector2/1 -> Product1/2
  Selector3/1 -> Product1/1
  Selector/1 -> Product2/2
  Selector1/1 -> Product2/1
  Vxyz/1 -> Selector3/1, Selector/1

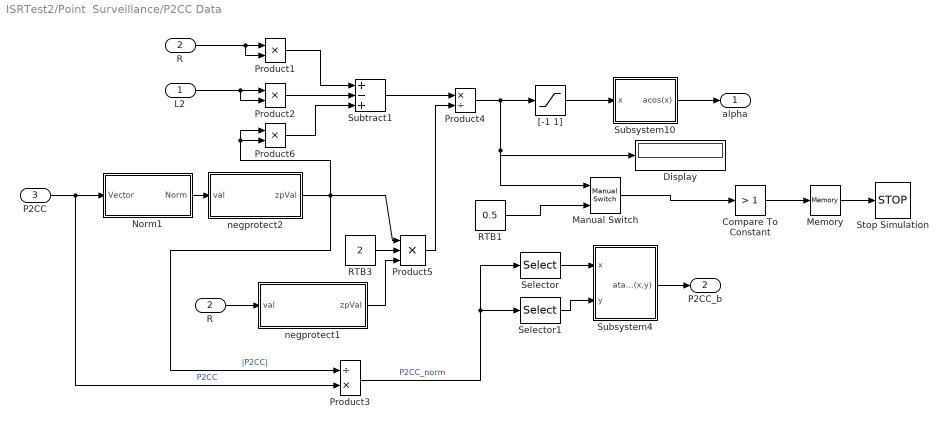
== system ISRTest2/Point  Surveillance/P2CC Data ==
  L2 : Inport
  R : Inport  Port=2
  P2CC : Inport  Port=3
  Compare To Constant : simulink/Logic and Bit Operations/Compare To Constant  SystemSampleTime=-1  relop=>  const=1  LogicOutDataTypeMode=boolean  ZeroCross=off
  Display : Display
  Manual Switch : simulink/Signal Routing/Manual Switch  SystemSampleTime=-1  sw=0  action=0  varsize=off
  Memory : Memory
  Norm1 : Subsystem
  Product1 : Product  RndMeth=Zero
  Product2 : Product  RndMeth=Zero
  Product3 : Product  Inputs=/*  RndMeth=Zero
  Product4 : Product  Inputs=*/  RndMeth=Zero
  Product5 : Product  Inputs=3  RndMeth=Zero
  Product6 : Product  RndMeth=Zero
  "R " : InportShadow  Port=2  LatchByCopyingInsideSignal=off
  RTB1 : Constant  Value=0.5  OutDataTypeMode=single
  RTB3 : Constant  Value=2  OutDataTypeMode=single
  Selector : Selector  IndexOptions=Index vector (dialog)  Indices=[2]  OutputSizes=1  InputPortWidth=3
  Selector1 : Selector  IndexOptions=Index vector (dialog)  Indices=[1]  OutputSizes=1  InputPortWidth=3
  Stop Simulation : Stop
  Subsystem10 : Subsystem
  Subsystem4 : Subsystem
  Subtract1 : Sum  Inputs=+-+  OutScaling=2^-10
  "[-1 1]" : Saturate  UpperLimit=1  LowerLimit=-1
  negprotect1 : Stateflow chart
  negprotect2 : Stateflow chart
  alpha : Outport
  P2CC_b : Outport  Port=2
  wires:
  "[-1 1]"/1 -> Subsystem10/1(x)
  Product6/1 -> Subtract1/3
  Selector1/1 -> Subsystem4/2(y)
  Selector/1 -> Subsystem4/1(x)
  Subsystem4/1(atan2(x,y)) -> P2CC_b/1
  Product3/1 -> Selector1/1, Selector/1  "P2CC_norm"
  negprotect2/1(zpVal) -> Product6/1, Product6/2, Product3/1, Product5/1  "|P2CC|"
  negprotect1/1(zpVal) -> Product5/3
  Subsystem10/1(acos(x)) -> alpha/1
  P2CC/1 -> Product3/2, Norm1/1(Vector)  "P2CC"
  Product4/1 -> "[-1 1]"/1, Display/1, Manual Switch/1
  Product5/1 -> Product4/2
  RTB3/1 -> Product5/2
  "R "/1 -> negprotect1/1(val)
  Subtract1/1 -> Product4/1
  Norm1/1(Norm) -> negprotect2/1(val)
  Product2/1 -> Subtract1/2
  Product1/1 -> Subtract1/1
  L2/1 -> Product2/2, Product2/1
  R/1 -> Product1/2, Product1/1
  Memory/1 -> Stop Simulation/1
  Compare To Constant/1 -> Memory/1
  Manual Switch/1 -> Compare To Constant/1
  RTB1/1 -> Manual Switch/2

== system ISRTest2/Point  Surveillance/Subsystem5 ==
  u : Inport
  Trigonometric Function : Trigonometry
  Trigonometric Function1 : Trigonometry  Operator=cos
  cos(u) : Outport
  sin(u) : Outport  Port=2
  wires:
  Trigonometric Function1/1 -> cos(u)/1
  u/1 -> Trigonometric Function/1, Trigonometric Function1/1
  Trigonometric Function/1 -> sin(u)/1

== system ISRTest2/Camera Track/Euler Angles to  Direction Cosine Matrix/A11 ==
  sin_cos : Inport
  Demux : Demux  Outputs=6
  Terminator{,1..3} (4 alike) : Terminator
  u(5)*u(6) : Product  RndMeth=Zero
  A11 : Outport
  wires:
  Demux/4 -> Terminator/1
  Demux/3 -> Terminator1/1
  Demux/5 -> u(5)*u(6)/1
  Demux/2 -> Terminator3/1
  Demux/1 -> Terminator2/1
  sin_cos/1 -> Demux/1
  u(5)*u(6)/1 -> A11/1
  Demux/6 -> u(5)*u(6)/2

== system ISRTest2/Camera Track/Euler Angles to  Direction Cosine Matrix/A12 ==
  sin_cos : Inport
  Demux : Demux  Outputs=6
  Terminator{,1..3} (4 alike) : Terminator
  u(3)*u(5) : Product  RndMeth=Zero
  A12 : Outport
  wires:
  Demux/6 -> Terminator1/1
  u(3)*u(5)/1 -> A12/1
  sin_cos/1 -> Demux/1
  Demux/1 -> Terminator2/1
  Demux/2 -> Terminator3/1
  Demux/5 -> u(3)*u(5)/2
  Demux/3 -> u(3)*u(5)/1
  Demux/4 -> Terminator/1

== system ISRTest2/Camera Track/Euler Angles to  Direction Cosine Matrix/A13 ==
  sin_cos : Inport
  Demux : Demux  Outputs=6
  Gain2 : Gain  Gain=-1  SaturateOnIntegerOverflow=on
  Terminator{,1..4} (5 alike) : Terminator
  A13 : Outport
  wires:
  Gain2/1 -> A13/1
  Demux/4 -> Terminator/1
  Demux/3 -> Terminator3/1
  Demux/5 -> Terminator4/1
  Demux/2 -> Gain2/1
  Demux/1 -> Terminator2/1
  sin_cos/1 -> Demux/1
  Demux/6 -> Terminator1/1

== system ISRTest2/Camera Track/Euler Angles to  Direction Cosine Matrix/A21 ==
  sin_cos : Inport
  Demux : Demux  Outputs=6
  Sum : Sum  Inputs=|+-
  Terminator : Terminator
  u(3)*u(4) : Product  RndMeth=Zero
  u(6)*u(1)*u(2) : Product  Inputs=3  RndMeth=Zero
  A21 : Outport
  wires:
  Demux/4 -> u(3)*u(4)/2
  Demux/3 -> u(3)*u(4)/1
  Demux/6 -> u(6)*u(1)*u(2)/1
  Demux/5 -> Terminator/1
  Demux/2 -> u(6)*u(1)*u(2)/3
  Demux/1 -> u(6)*u(1)*u(2)/2
  sin_cos/1 -> Demux/1
  u(6)*u(1)*u(2)/1 -> Sum/1
  u(3)*u(4)/1 -> Sum/2
  Sum/1 -> A21/1

== system ISRTest2/Camera Track/Euler Angles to  Direction Cosine Matrix/A22 ==
  sin_cos : Inport
  Demux : Demux  Outputs=6
  Sum : Sum  Inputs=|++
  Terminator : Terminator
  u(1)*u(2)*u(3) : Product  Inputs=3  RndMeth=Zero
  u(4)*u(6) : Product  RndMeth=Zero
  A22 : Outport
  wires:
  Demux/6 -> u(4)*u(6)/2
  Sum/1 -> A22/1
  u(4)*u(6)/1 -> Sum/2
  u(1)*u(2)*u(3)/1 -> Sum/1
  sin_cos/1 -> Demux/1
  Demux/1 -> u(1)*u(2)*u(3)/1
  Demux/2 -> u(1)*u(2)*u(3)/2
  Demux/5 -> Terminator/1
  Demux/3 -> u(1)*u(2)*u(3)/3
  Demux/4 -> u(4)*u(6)/1

== system ISRTest2/Camera Track/Euler Angles to  Direction Cosine Matrix/A23 ==
  sin_cos : Inport
  Demux : Demux  Outputs=6
  Terminator{,1..3} (4 alike) : Terminator
  u(1)*u(3) : Product  RndMeth=Zero
  A23 : Outport
  wires:
  Demux/4 -> Terminator/1
  Demux/3 -> Terminator2/1
  Demux/5 -> u(1)*u(3)/2
  Demux/2 -> Terminator3/1
  Demux/1 -> u(1)*u(3)/1
  sin_cos/1 -> Demux/1
  u(1)*u(3)/1 -> A23/1
  Demux/6 -> Terminator1/1

== system ISRTest2/Camera Track/Euler Angles to  Direction Cosine Matrix/A31 ==
  sin_cos : Inport
  Demux : Demux  Outputs=6
  Sum : Sum  Inputs=|++
  Terminator : Terminator
  u(1)*u(3) : Product  RndMeth=Zero
  u(2)*u(4)*u(6) : Product  Inputs=3  RndMeth=Zero
  A31 : Outport
  wires:
  u(1)*u(3)/1 -> Sum/1
  Demux/6 -> u(2)*u(4)*u(6)/3
  Sum/1 -> A31/1
  u(2)*u(4)*u(6)/1 -> Sum/2
  sin_cos/1 -> Demux/1
  Demux/1 -> u(1)*u(3)/1
  Demux/2 -> u(2)*u(4)*u(6)/1
  Demux/5 -> Terminator/1
  Demux/3 -> u(1)*u(3)/2
  Demux/4 -> u(2)*u(4)*u(6)/2

== system ISRTest2/Camera Track/Euler Angles to  Direction Cosine Matrix/A32 ==
  sin_cos : Inport
  Demux : Demux  Outputs=6
  Sum : Sum  Inputs=|+-
  Terminator : Terminator
  u(1)*u(6) : Product  RndMeth=Zero
  u(2)*u(3)*u(4) : Product  Inputs=3  RndMeth=Zero
  A32 : Outport
  wires:
  Demux/4 -> u(2)*u(3)*u(4)/3
  Demux/3 -> u(2)*u(3)*u(4)/2
  Demux/5 -> Terminator/1
  Demux/2 -> u(2)*u(3)*u(4)/1
  Demux/1 -> u(1)*u(6)/2
  sin_cos/1 -> Demux/1
  u(2)*u(3)*u(4)/1 -> Sum/1
  u(1)*u(6)/1 -> Sum/2
  Sum/1 -> A32/1
  Demux/6 -> u(1)*u(6)/1

== system ISRTest2/Camera Track/Euler Angles to  Direction Cosine Matrix/A33 ==
  sin_cos : Inport
  Demux : Demux  Outputs=6
  Terminator{,1..3} (4 alike) : Terminator
  u(4)*u(5) : Product  RndMeth=Zero
  A33 : Outport
  wires:
  Demux/6 -> Terminator/1
  u(4)*u(5)/1 -> A33/1
  sin_cos/1 -> Demux/1
  Demux/1 -> Terminator2/1
  Demux/2 -> Terminator3/1
  Demux/5 -> u(4)*u(5)/2
  Demux/3 -> Terminator1/1
  Demux/4 -> u(4)*u(5)/1

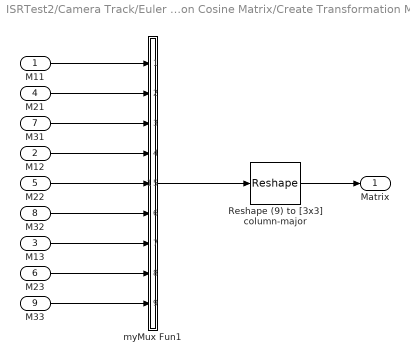
== system ISRTest2/Camera Track/Euler Angles to  Direction Cosine Matrix/Create Transformation Matrix ==
  M11 : Inport
  M12 : Inport  Port=2
  M13 : Inport  Port=3
  M21 : Inport  Port=4
  M22 : Inport  Port=5
  M23 : Inport  Port=6
  M31 : Inport  Port=7
  M32 : Inport  Port=8
  M33 : Inport  Port=9
  Reshape (9) to [3x3] column-major : Reshape  OutputDimensionality=Customize  OutputDimensions=[3,3]
  myMux Fun1 : Stateflow chart
  Matrix : Outport
  wires:
  M33/1 -> myMux Fun1/9(u9)
  M23/1 -> myMux Fun1/8(u8)
  M13/1 -> myMux Fun1/7(u7)
  M32/1 -> myMux Fun1/6(u6)
  Reshape (9) to [3x3] column-major/1 -> Matrix/1
  M22/1 -> myMux Fun1/5(u5)
  M12/1 -> myMux Fun1/4(u4)
  M31/1 -> myMux Fun1/3(u3)
  M21/1 -> myMux Fun1/2(u2)
  M11/1 -> myMux Fun1/1(u1)
  myMux Fun1/1(y) -> Reshape (9) to [3x3] column-major/1

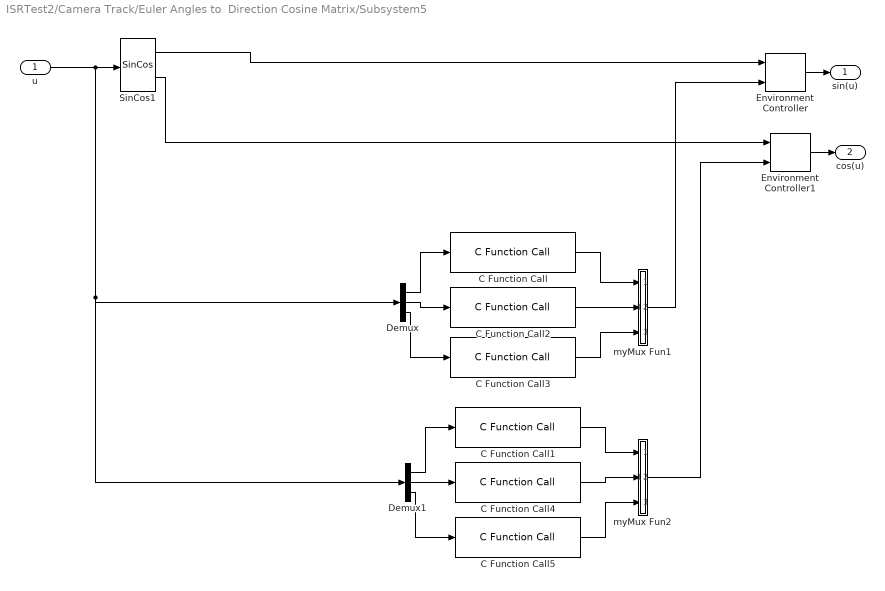
== system ISRTest2/Camera Track/Euler Angles to  Direction Cosine Matrix/Subsystem5 ==
  u : Inport
  C Function Call : dsPICdrivers/OTHERS/C Function Call  Tag=dsPIC_dsPIC_CFunctionCall  fctName='mySin'  INPUT_SIZE=1  INPUT1=real32  INPUT2=--  INPUT3=--  OUTPUT_SIZE=1  OUTPUT1=real32  SampleTime=-1  InputType=[ 7 ]  OutputType=[ 7 ]  FctDeclaration=extern real32_T mySin(real32_T u1);  FctCall=%y1 = mySin(%u1);  OrderingInOutPopup=None
  C Function Call1 : dsPICdrivers/OTHERS/C Function Call  Tag=dsPIC_dsPIC_CFunctionCall  fctName='myCos'  INPUT_SIZE=1  INPUT1=real32  INPUT2=--  INPUT3=--  OUTPUT_SIZE=1  OUTPUT1=real32  SampleTime=-1  InputType=[ 7 ]  OutputType=[ 7 ]  FctDeclaration=extern real32_T myCos(real32_T u1);  FctCall=%y1 = myCos(%u1);  OrderingInOutPopup=None
  C Function Call2 : dsPICdrivers/OTHERS/C Function Call  Tag=dsPIC_dsPIC_CFunctionCall  fctName='mySin'  INPUT_SIZE=1  INPUT1=real32  INPUT2=--  INPUT3=--  OUTPUT_SIZE=1  OUTPUT1=real32  SampleTime=-1  InputType=[ 7 ]  OutputType=[ 7 ]  FctDeclaration=extern real32_T mySin(real32_T u1);  FctCall=%y1 = mySin(%u1);  OrderingInOutPopup=None
  C Function Call3 : dsPICdrivers/OTHERS/C Function Call  Tag=dsPIC_dsPIC_CFunctionCall  fctName='mySin'  INPUT_SIZE=1  INPUT1=real32  INPUT2=--  INPUT3=--  OUTPUT_SIZE=1  OUTPUT1=real32  SampleTime=-1  InputType=[ 7 ]  OutputType=[ 7 ]  FctDeclaration=extern real32_T mySin(real32_T u1);  FctCall=%y1 = mySin(%u1);  OrderingInOutPopup=None
  C Function Call4 : dsPICdrivers/OTHERS/C Function Call  Tag=dsPIC_dsPIC_CFunctionCall  fctName='myCos'  INPUT_SIZE=1  INPUT1=real32  INPUT2=--  INPUT3=--  OUTPUT_SIZE=1  OUTPUT1=real32  SampleTime=-1  InputType=[ 7 ]  OutputType=[ 7 ]  FctDeclaration=extern real32_T myCos(real32_T u1);  FctCall=%y1 = myCos(%u1);  OrderingInOutPopup=None
  C Function Call5 : dsPICdrivers/OTHERS/C Function Call  Tag=dsPIC_dsPIC_CFunctionCall  fctName='myCos'  INPUT_SIZE=1  INPUT1=real32  INPUT2=--  INPUT3=--  OUTPUT_SIZE=1  OUTPUT1=real32  SampleTime=-1  InputType=[ 7 ]  OutputType=[ 7 ]  FctDeclaration=extern real32_T myCos(real32_T u1);  FctCall=%y1 = myCos(%u1);  OrderingInOutPopup=None
  Demux : Demux  Outputs=3
  Demux1 : Demux  Outputs=3
  Environment Controller : simulink/Signal Routing/Environment Controller  SystemSampleTime=-1
  Environment Controller1 : simulink/Signal Routing/Environment Controller  SystemSampleTime=-1
  SinCos1 : aerolibutil/SinCos  SystemSampleTime=-1
  myMux Fun1 : Stateflow chart
  myMux Fun2 : Stateflow chart
  sin(u) : Outport
  cos(u) : Outport  Port=2
  wires:
  myMux Fun2/1(y) -> Environment Controller1/2
  myMux Fun1/1(y) -> Environment Controller/2
  Demux1/3 -> C Function Call5/1
  Demux1/2 -> C Function Call4/1
  Demux1/1 -> C Function Call1/1
  Demux/3 -> C Function Call3/1
  Demux/2 -> C Function Call2/1
  Demux/1 -> C Function Call/1
  C Function Call5/1 -> myMux Fun2/3(u3)
  C Function Call4/1 -> myMux Fun2/2(u2)
  C Function Call1/1 -> myMux Fun2/1(u1)
  C Function Call3/1 -> myMux Fun1/3(u3)
  C Function Call2/1 -> myMux Fun1/2(u2)
  C Function Call/1 -> myMux Fun1/1(u1)
  SinCos1/2 -> Environment Controller1/1
  Environment Controller1/1 -> cos(u)/1
  u/1 -> Demux1/1, Demux/1, SinCos1/1
  SinCos1/1 -> Environment Controller/1
  Environment Controller/1 -> sin(u)/1

== system ISRTest2/Camera Track/Norm/Subsystem1 ==
  x : Inport
  C Function Call : S-Function  Tag=dsPIC_dsPIC_CFunctionCall  FunctionName=dsPIC_C_function_Call  Parameters=INPUT_SIZE,OUTPUT_SIZE,InputType,OutputType,SampleTime,fOrderingInOut  mask(C Function Call){fctName='mySqrt', INPUT_SIZE=1, INPUT1=real32, INPUT2=--, INPUT3=--, OUTPUT_SIZE=1, OUTPUT1=real32, SampleTime=-1, InputType=[ 7 ], OutputType=[ 7 ], FctDeclaration=extern real32_T mySqrt(real32_T u1);, FctCall=%y1 = mySqrt(%u1);, OrderingInOutPopup=None}
      mask prompts: fctName "Function Name"; INPUT_SIZE "Global Input Size"; INPUT1 "Input 1"; INPUT2 "Input 2"; INPUT3 "Input 3"; OUTPUT_SIZE "Output size"; OUTPUT1 "Output type"; InputType "NbrInput"; OutputType "NbrOutput"; FctDeclaration "Function Declaration :"; FctCall "Function Call :"; OrderingInOutPopup "Block Ordering Input / Output"
      mask help: call user defined C function
      mask init:
      | dsPIC_C_function_Call_callback();
      mask Help: http://www.kerhuel.eu/wiki/index.php5?title=Block/C_Function_Call#1
      mask StyleString: edit,edit,popup(--|int8|uint8|int16|uint16|int32|uint32|real32|real64),popup(--|int8|uint8|int16|uint16|int32|uint32|real32|real64),popup(--|int8|uint8|int16|uint16|int32|uint32|real32|real64),edit,popup(--|int8|uint8|int16|uint16|int32|uint32|real32|real64),edit,edit,edit,edit,edit,popup(None|Input|Output|Input & Output)
      mask CallbackString:
      | dsPIC_C_function_Call_callback();|dsPIC_C_function_Call_callback();|dsPIC_C_function_Call_callback();|dsPIC_C_function_Call_callback();
      | |dsPIC_C_function_Call_callback();|dsPIC_C_function_Call_callback();|dsPIC_C_function_Call_callback();|dsPIC_C_function_Call_callback();|||% for information only|% for information only|
      mask Display:
      | fprintf('C function call\nmySqrt');
      | port_label('input',1,' u1');
      | port_label('output',1,'y');
  Environment Controller : Subsystem  mask(Environment Controller){}
      mask help: Output the simulation (Sim) or Real-Time Workshop (RTW) port depending on the current environment. With optimizations enabled, unnecessary blocks leading to the unused port are not executed. Both input signals must be the same width.
      mask init:
      | switch_mode = rtwenvironmentmode(bdroot(gcbh));
  Math Function1 : Math  Operator=sqrt  SaturateOnIntegerOverflow=on
  negprotect : Stateflow chart
  sqrt(x) : Outport
  wires:
  x/1 -> negprotect/1(val)
  negprotect/1(zpVal) -> Math Function1/1, C Function Call/1
  Environment Controller/1(Out) -> sqrt(x)/1
  Math Function1/1 -> Environment Controller/1(Sim)
  C Function Call/1 -> Environment Controller/2(RTW)

== system ISRTest2/Camera Track/Norm/Subsystem3 ==
  x : Inport
  y : Inport  Port=2
  Dot Product : simulink/Math Operations/Dot Product  InputSameDT=on  OutDataType=sfix(16)  OutScaling=2^-10  DoSatur=off
  Embedded MATLAB Function : Stateflow chart
  Environment Controller : simulink/Signal Routing/Environment Controller  SystemSampleTime=-1
  x dot y : Outport
  wires:
  Environment Controller/1 -> x dot y/1
  Embedded MATLAB Function/1(xDoty) -> Environment Controller/2
  Dot Product/1 -> Environment Controller/1
  x/1 -> Dot Product/1, Embedded MATLAB Function/1(x)
  y/1 -> Dot Product/2, Embedded MATLAB Function/2(y)

== system ISRTest2/Camera Track/Norm1/Subsystem1 ==
  x : Inport
  C Function Call : S-Function  Tag=dsPIC_dsPIC_CFunctionCall  FunctionName=dsPIC_C_function_Call  Parameters=INPUT_SIZE,OUTPUT_SIZE,InputType,OutputType,SampleTime,fOrderingInOut  mask(C Function Call){fctName='mySqrt', INPUT_SIZE=1, INPUT1=real32, INPUT2=--, INPUT3=--, OUTPUT_SIZE=1, OUTPUT1=real32, SampleTime=-1, InputType=[ 7 ], OutputType=[ 7 ], FctDeclaration=extern real32_T mySqrt(real32_T u1);, FctCall=%y1 = mySqrt(%u1);, OrderingInOutPopup=None}
      mask prompts: fctName "Function Name"; INPUT_SIZE "Global Input Size"; INPUT1 "Input 1"; INPUT2 "Input 2"; INPUT3 "Input 3"; OUTPUT_SIZE "Output size"; OUTPUT1 "Output type"; InputType "NbrInput"; OutputType "NbrOutput"; FctDeclaration "Function Declaration :"; FctCall "Function Call :"; OrderingInOutPopup "Block Ordering Input / Output"
      mask help: call user defined C function
      mask init:
      | dsPIC_C_function_Call_callback();
      mask Help: http://www.kerhuel.eu/wiki/index.php5?title=Block/C_Function_Call#1
      mask StyleString: edit,edit,popup(--|int8|uint8|int16|uint16|int32|uint32|real32|real64),popup(--|int8|uint8|int16|uint16|int32|uint32|real32|real64),popup(--|int8|uint8|int16|uint16|int32|uint32|real32|real64),edit,popup(--|int8|uint8|int16|uint16|int32|uint32|real32|real64),edit,edit,edit,edit,edit,popup(None|Input|Output|Input & Output)
      mask CallbackString:
      | dsPIC_C_function_Call_callback();|dsPIC_C_function_Call_callback();|dsPIC_C_function_Call_callback();|dsPIC_C_function_Call_callback();
      | |dsPIC_C_function_Call_callback();|dsPIC_C_function_Call_callback();|dsPIC_C_function_Call_callback();|dsPIC_C_function_Call_callback();|||% for information only|% for information only|
      mask Display:
      | fprintf('C function call\nmySqrt');
      | port_label('input',1,' u1');
      | port_label('output',1,'y');
  Environment Controller : Subsystem  mask(Environment Controller){}
      mask help: Output the simulation (Sim) or Real-Time Workshop (RTW) port depending on the current environment. With optimizations enabled, unnecessary blocks leading to the unused port are not executed. Both input signals must be the same width.
      mask init:
      | switch_mode = rtwenvironmentmode(bdroot(gcbh));
  Math Function1 : Math  Operator=sqrt  SaturateOnIntegerOverflow=on
  negprotect : Stateflow chart
  sqrt(x) : Outport
  wires:
  C Function Call/1 -> Environment Controller/2(RTW)
  Math Function1/1 -> Environment Controller/1(Sim)
  Environment Controller/1(Out) -> sqrt(x)/1
  negprotect/1(zpVal) -> C Function Call/1, Math Function1/1
  x/1 -> negprotect/1(val)

== system ISRTest2/Camera Track/Norm1/Subsystem3 ==
  x : Inport
  y : Inport  Port=2
  Dot Product : simulink/Math Operations/Dot Product  InputSameDT=on  OutDataType=sfix(16)  OutScaling=2^-10  DoSatur=off
  Embedded MATLAB Function : Stateflow chart
  Environment Controller : simulink/Signal Routing/Environment Controller  SystemSampleTime=-1
  x dot y : Outport
  wires:
  y/1 -> Embedded MATLAB Function/2(y), Dot Product/2
  x/1 -> Embedded MATLAB Function/1(x), Dot Product/1
  Dot Product/1 -> Environment Controller/1
  Embedded MATLAB Function/1(xDoty) -> Environment Controller/2
  Environment Controller/1 -> x dot y/1
